simulink model "dynamic_simulation_control_for_id"  (R2017b)
settings: Solver=FixedStepAuto  StartTime=0.0  StopTime=60.0  FixedStep=dt  RelTol=1e-3
values from neighbouring files (symbols this model uses):
  dth0 = [0; 0; 0]    [dynamic_simulation.m]    (also in init_dynamic_sim.m = dq0)
  Fv = zeros(3,3)    [DynModel_3DOF.m]    (also in InvDynModel_3DOF.m; init_dynamic_sim.m = diag([0.5,0.37,0.7]))
  fz0 = 0    [init_dynamic_sim.m]
  K = 0.015    [init_dynamic_sim.m]
  Ki = 0.08    [init_dynamic_sim.m]
  Kj = [1;1;1]*5    [init_dynamic_sim.m]
  Kjd = [1;1;1]*0.1    [init_dynamic_sim.m]
  Kv = [2500;1500;2000]/256    [init_dynamic_sim.m]
  Kvi = [3000;900;1000]/65536    [init_dynamic_sim.m]
  Kx = [20;0;0]    [init_dynamic_sim.m]
  Kxi = [0;0;0]    [init_dynamic_sim.m]
  nu = nu.*eye(3)    [DynModel_3DOF.m]    (also in InvDynModel_3DOF.m; init_dynamic_sim.m = 0.1)
  th0 = 0    [DGM_youBot.m]    (also in DGM_youBot_sym.m; dynamic_simulation.m = q_dh - (q0_kuka - q_rob); init_dynamic_sim.m = theta_DH(2:4) - (q0 - KUKA_offset(2:4)))
  thmax = theta_DH - (qmin - KUKA_offset)    [init_dynamic_sim.m]
  thmin = theta_DH - (qmax - KUKA_offset)    [init_dynamic_sim.m]
undefined symbols (not defined in the file or in its folder): p0
settings Model: Creator=fortineau_vin  LastModifiedBy=fortineau_vin

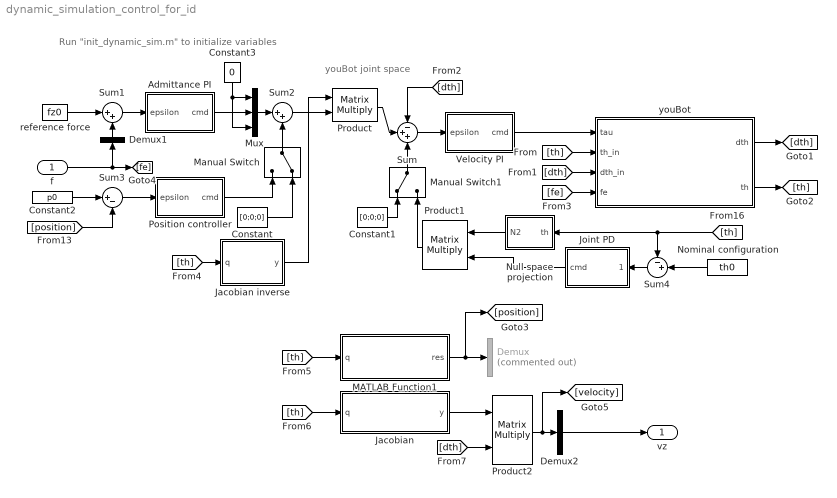
== system dynamic_simulation_control_for_id ==
  note: Run "init_dynamic_sim.m" to initialize variables
  note: youBot joint space
  f : Inport
  Admittance PI : Subsystem
  Constant : Constant  Value=[0;0;0]
  Constant1 : Constant  Value=[0;0;0]
  Constant2 : Constant  Value=p0
  Constant3 : Constant  Value=0
  Demux : Demux  Commented=on  Outputs=3
  Demux1 : Demux  Outputs=3
  Demux2 : Demux  Outputs=3
  Jacobian : MATLAB Function  TreatAsAtomicUnit=on
  Jacobian inverse : MATLAB Function  TreatAsAtomicUnit=on
  Joint PD : Subsystem
  MATLAB Function1 : MATLAB Function  TreatAsAtomicUnit=on
  Manual Switch : ManualSwitch  CurrentSetting=0
  Manual Switch1 : ManualSwitch
  Mux : Mux  Inputs=3
  Nominal configuration : Constant  Value=th0
  Null space projection : Subsystem
  Position controller : Subsystem
  Product : Product  Multiplication=Matrix(*)
  Product1 : Product  Multiplication=Matrix(*)
  Product2 : Product  Multiplication=Matrix(*)
  Sum : Sum  Inputs=-++
  Sum1 : Sum  Inputs=|++
  Sum2 : Sum  Inputs=|++
  Sum3 : Sum  Inputs=|+-
  Sum4 : Sum  Inputs=-+|
  Velocity PI : Subsystem
  reference force : Constant  Value=fz0
  youBot : Subsystem
  vz : Outport
  wires:
  Sum/1 -> Velocity PI/1(epsilon)
  [dth] -> Sum/1
  Product/1 -> Sum/2
  Sum1/1 -> Admittance PI/1(epsilon)
  [th] -> Jacobian inverse/1(q)
  Sum3/1 -> Position controller/1(epsilon)
  Constant2/1 -> Sum3/1
  [position] -> Sum3/2
  Admittance PI/1(cmd) -> Mux/2
  Mux/1 -> Sum2/1
  Constant3/1 -> Mux/3, Mux/1
  reference force/1 -> Sum1/1
  [th] -> youBot/2(th_in)
  [dth] -> youBot/3(dth_in)
  [fe] -> youBot/4(fe)
  youBot/1(dth) -> [dth]
  youBot/2(th) -> [th]
  Sum4/1 -> Joint PD/1(epsilon)
  Nominal configuration/1 -> Sum4/2
  Null space projection/1(N2) -> Product1/1
  [th] -> Null space projection/1(th), Sum4/1
  Joint PD/1(cmd) -> Product1/2
  Sum2/1 -> Product/2
  Jacobian inverse/1(y) -> Product/1
  Velocity PI/1(cmd) -> youBot/1(tau)
  [th] -> MATLAB Function1/1(q)
  MATLAB Function1/1(res) -> [position], Demux/1
  Demux1/2 -> Sum1/2
  f/1 -> [fe], Demux1/1
  Position controller/1(cmd) -> Manual Switch/1
  Manual Switch/1 -> Sum2/2
  Constant/1 -> Manual Switch/2
  Product1/1 -> Manual Switch1/2
  Manual Switch1/1 -> Sum/3
  Constant1/1 -> Manual Switch1/1
  [th] -> Jacobian/1(q)
  Jacobian/1(y) -> Product2/1
  [dth] -> Product2/2
  Demux2/2 -> vz/1
  Product2/1 -> [velocity], Demux2/1

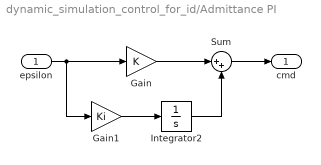
== system dynamic_simulation_control_for_id/Admittance PI ==
  epsilon : Inport
  Gain : Gain  Gain=K
  Gain1 : Gain  Gain=Ki
  Integrator2 : Integrator
  Sum : Sum  Inputs=|++
  cmd : Outport
  wires:
  Integrator2/1 -> Sum/2
  Gain/1 -> Sum/1
  Gain1/1 -> Integrator2/1
  epsilon/1 -> Gain/1, Gain1/1
  Sum/1 -> cmd/1

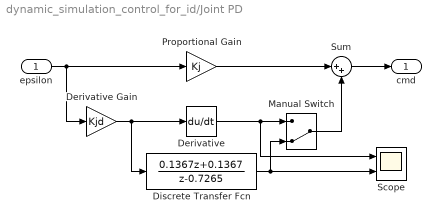
== system dynamic_simulation_control_for_id/Joint PD ==
  epsilon : Inport
  " Derivative Gain" : Gain  Gain=Kjd
  Derivative : Derivative
  Discrete Transfer Fcn : DiscreteTransferFcn  Numerator=[0.1367 0.1367]  Denominator=[1 -0.7265]
  Manual Switch : ManualSwitch  CurrentSetting=0
  Proportional Gain : Gain  Gain=Kj
  Scope : Scope  NumInputPorts=2
  Sum : Sum  Inputs=|++
  cmd : Outport
  wires:
  Sum/1 -> cmd/1
  epsilon/1 -> " Derivative Gain"/1, Proportional Gain/1
  " Derivative Gain"/1 -> Derivative/1, Discrete Transfer Fcn/1
  Proportional Gain/1 -> Sum/1
  Derivative/1 -> Scope/1, Manual Switch/1
  Manual Switch/1 -> Sum/2
  Discrete Transfer Fcn/1 -> Scope/2, Manual Switch/2

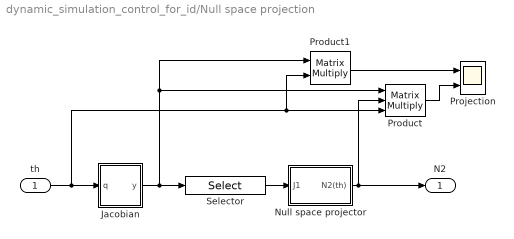
== system dynamic_simulation_control_for_id/Null space projection ==
  th : Inport
  Jacobian : MATLAB Function  TreatAsAtomicUnit=on
  Null space projector : Subsystem
  Product : Product  Inputs=3  Multiplication=Matrix(*)
  Product1 : Product  Multiplication=Matrix(*)
  Projection : Scope  NumInputPorts=2
  Selector : Selector  NumberOfDimensions=2  InputPortWidth=3  IndexOptions=Index vector (dialog),Index vector (dialog)  Indices=2,[1 2 3]  OutputSizes=1,1
  N2 : Outport
  wires:
  Null space projector/1(N2(th)) -> N2/1, Product/2
  Jacobian/1(y) -> Product1/1, Product/1, Selector/1
  Selector/1 -> Null space projector/1(J1)
  th/1 -> Product1/2, Product/3, Jacobian/1(q)
  Product/1 -> Projection/2
  Product1/1 -> Projection/1

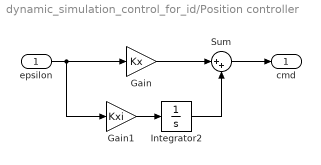
== system dynamic_simulation_control_for_id/Position controller ==
  epsilon : Inport
  Gain : Gain  Gain=Kx
  Gain1 : Gain  Gain=Kxi
  Integrator2 : Integrator
  Sum : Sum  Inputs=|++
  cmd : Outport
  wires:
  Sum/1 -> cmd/1
  epsilon/1 -> Gain1/1, Gain/1
  Gain1/1 -> Integrator2/1
  Gain/1 -> Sum/1
  Integrator2/1 -> Sum/2

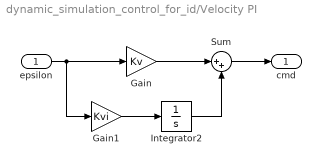
== system dynamic_simulation_control_for_id/Velocity PI ==
  epsilon : Inport
  Gain : Gain  Gain=Kv
  Gain1 : Gain  Gain=Kvi
  Integrator2 : Integrator
  Sum : Sum  Inputs=|++
  cmd : Outport
  wires:
  Sum/1 -> cmd/1
  epsilon/1 -> Gain1/1, Gain/1
  Gain1/1 -> Integrator2/1
  Gain/1 -> Sum/1
  Integrator2/1 -> Sum/2

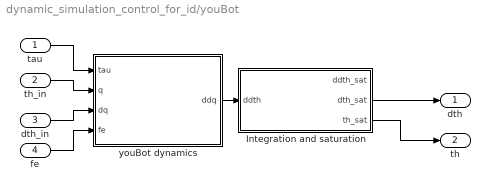
== system dynamic_simulation_control_for_id/youBot ==
  tau : Inport
  th_in : Inport  Port=2
  dth_in : Inport  Port=3
  fe : Inport  Port=4
  Integration and saturation : Subsystem
  youBot dynamics : Subsystem
  dth : Outport
  th : Outport  Port=2
  wires:
  tau/1 -> youBot dynamics/1(tau)
  youBot dynamics/1(ddq) -> Integration and saturation/1(ddth)
  dth_in/1 -> youBot dynamics/3("dq ")
  th_in/1 -> youBot dynamics/2("q ")
  fe/1 -> youBot dynamics/4(fe)
  Integration and saturation/3(th_sat) -> th/1
  Integration and saturation/2(dth_sat) -> dth/1

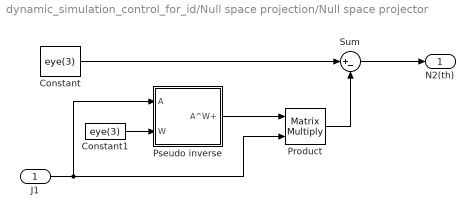
== system dynamic_simulation_control_for_id/Null space projection/Null space projector ==
  J1 : Inport
  Constant : Constant  Value=eye(3)  VectorParams1D=off
  Constant1 : Constant  Value=eye(3)  VectorParams1D=off
  Product : Product  Multiplication=Matrix(*)
  Pseudo inverse : Subsystem
  Sum : Sum  Inputs=|+-
  N2(th) : Outport
  wires:
  Constant/1 -> Sum/1
  Constant1/1 -> Pseudo inverse/2(W)
  J1/1 -> Pseudo inverse/1(A), Product/2
  Pseudo inverse/1(A^W+) -> Product/1
  Product/1 -> Sum/2
  Sum/1 -> N2(th)/1

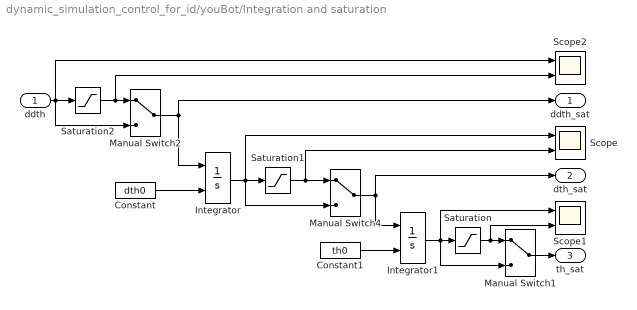
== system dynamic_simulation_control_for_id/youBot/Integration and saturation ==
  ddth : Inport
  Constant : Constant  Value=dth0
  Constant1 : Constant  Value=th0
  Integrator : Integrator  InitialConditionSource=external
  Integrator1 : Integrator  InitialConditionSource=external
  Manual Switch1 : ManualSwitch
  Manual Switch2 : ManualSwitch
  Manual Switch4 : ManualSwitch
  Saturation : Saturate  UpperLimit=thmax(2:4)'  LowerLimit=thmin(2:4)'
  Saturation1 : Saturate  UpperLimit=[2.685122; 4.188790; 5.899705]  LowerLimit=[-2.685122; -4.188790; -5.899705]
  Saturation2 : Saturate  UpperLimit=[10;10;10]  LowerLimit=[-10;-10;-10]
  Scope : Scope  NumInputPorts=2
  Scope1 : Scope  NumInputPorts=2
  Scope2 : Scope  NumInputPorts=2
  ddth_sat : Outport
  dth_sat : Outport  Port=2
  th_sat : Outport  Port=3
  wires:
  Manual Switch2/1 -> ddth_sat/1, Integrator/1
  Manual Switch1/1 -> th_sat/1
  Manual Switch4/1 -> Integrator1/1, dth_sat/1
  ddth/1 -> Scope2/1, Manual Switch2/2, Saturation2/1
  Saturation2/1 -> Scope2/2, Manual Switch2/1
  Saturation1/1 -> Scope/2, Manual Switch4/1
  Saturation/1 -> Scope1/2, Manual Switch1/1
  Constant/1 -> Integrator/2
  Integrator/1 -> Scope/1, Manual Switch4/2, Saturation1/1
  Integrator1/1 -> Scope1/1, Manual Switch1/2, Saturation/1
  Constant1/1 -> Integrator1/2

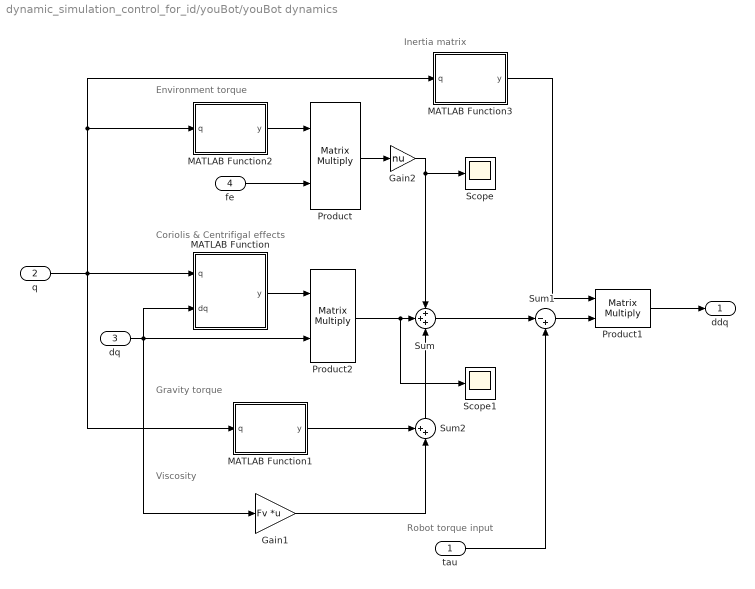
== system dynamic_simulation_control_for_id/youBot/youBot dynamics ==
  note: Coriolis & Centrifigal effects
  note: Gravity torque
  note: Environment torque
  note: Robot torque input
  note: Inertia matrix
  note: Viscosity
  tau : Inport
  "q " : Inport  Port=2
  "dq " : Inport  Port=3
  fe : Inport  Port=4
  Gain1 : Gain  Gain=Fv  Multiplication=Matrix(K*u)
  Gain2 : Gain  Gain=nu
  MATLAB Function : MATLAB Function  TreatAsAtomicUnit=on
  MATLAB Function1 : MATLAB Function  TreatAsAtomicUnit=on
  MATLAB Function2 : MATLAB Function  TreatAsAtomicUnit=on
  MATLAB Function3 : MATLAB Function  TreatAsAtomicUnit=on
  Product : Product  Multiplication=Matrix(*)
  Product1 : Product  Multiplication=Matrix(*)
  Product2 : Product  Multiplication=Matrix(*)
  Scope : Scope
  Scope1 : Scope
  Sum : Sum  Inputs=+++
  Sum1 : Sum  Inputs=|-+
  Sum2 : Sum  Inputs=++|
  ddq : Outport
  wires:
  "dq "/1 -> Gain1/1, Product2/2, MATLAB Function/2(dq)
  "q "/1 -> MATLAB Function3/1(q), MATLAB Function2/1(q), MATLAB Function1/1(q), MATLAB Function/1(q)
  Product/1 -> Gain2/1
  Product1/1 -> ddq/1
  Sum/1 -> Sum1/1
  tau/1 -> Sum1/2
  Product2/1 -> Scope1/1, Sum/2
  MATLAB Function/1(y) -> Product2/1
  MATLAB Function2/1(y) -> Product/1
  fe/1 -> Product/2
  MATLAB Function3/1(y) -> Product1/1
  Sum1/1 -> Product1/2
  Gain2/1 -> Scope/1, Sum/1
  MATLAB Function1/1(y) -> Sum2/1
  Sum2/1 -> Sum/3
  Gain1/1 -> Sum2/2

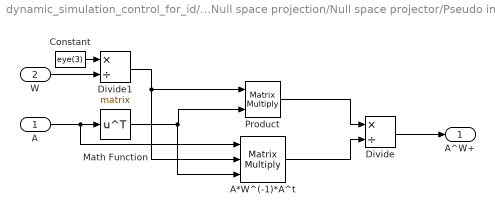
== system dynamic_simulation_control_for_id/Null space projection/Null space projector/Pseudo inverse ==
  A : Inport
  W : Inport  Port=2
  A*W^(-1)*A^t : Product  Inputs=3  Multiplication=Matrix(*)
  Constant : Constant  Value=eye(3)
  Divide : Product  Inputs=*/
  Divide1 : Product  Inputs=*/  Multiplication=Matrix(*)
  Math Function : Math  Operator=transpose  SaturateOnIntegerOverflow=on
  Product : Product  Multiplication=Matrix(*)
  A^W+ : Outport
  wires:
  W/1 -> Divide1/2
  A/1 -> A*W^(-1)*A^t/1, Math Function/1
  Math Function/1 -> A*W^(-1)*A^t/3, Product/2
  Divide1/1 -> A*W^(-1)*A^t/2, Product/1
  Product/1 -> Divide/1
  A*W^(-1)*A^t/1 -> Divide/2
  Divide/1 -> A^W+/1
  Constant/1 -> Divide1/1

== matlab function dynamic_simulation_control_for_id/youBot/youBot dynamics/MATLAB Function1 ==
  data: q input; y output
function y = G_sim(q)
q1 = q(1);
q2 = q(2);
q3 = q(3);
y = G_3DOF(q1,q2,q3);

== matlab function dynamic_simulation_control_for_id/youBot/youBot dynamics/MATLAB Function ==
  data: q input; y output; dq input
function y = C_sim(q,dq)
q2 = q(2);
q3 = q(3);
dq1 = dq(1);
dq2 = dq(2);
dq3 = dq(3);
y = C_3DOF(dq1,dq2,dq3,q2,q3);

== matlab function dynamic_simulation_control_for_id/youBot/youBot dynamics/MATLAB Function2 ==
  data: q input; y output
function y = tJ_sim(q)
q1 = q(1);
q2 = q(2);
q3 = q(3);
y = J0E_3DOF(q1,q2,q3)';

== matlab function dynamic_simulation_control_for_id/youBot/youBot dynamics/MATLAB Function3 ==
  data: q input; y output
function y = iM_sim(q)
q2 = q(2);
q3 = q(3);
y = iM_3DOF(q2,q3);

== matlab function dynamic_simulation_control_for_id/Jacobian inverse ==
  data: q input; y output
function y = iJ(q)
q1 = q(1);
q2 = q(2);
q3 = q(3);
y = iJ0E_3DOF(q1,q2,q3);

== matlab function dynamic_simulation_control_for_id/Jacobian ==
  data: q input; y output
function y = J(q)
q1 = q(1);
q2 = q(2);
q3 = q(3);
y = J0E_3DOF(q1,q2,q3);

== matlab function dynamic_simulation_control_for_id/Null space projection/Jacobian ==
  data: q input; y output
function y = J(q)
q1 = q(1);
q2 = q(2);
q3 = q(3);
y = J0E_3DOF(q1,q2,q3);

== matlab function dynamic_simulation_control_for_id/MATLAB Function1 ==
  data: q input; res output
function res = forwardKinematics(q)

x0 = 0;
le = 0.1;

[p,r,~] = DGM_youBot(q, x0, le);

x  = p(1);
z  = p(3);
ry = acos(r(1,1));

res = [x,z,ry]';
